simulink model "updated_target_driver_2026_withVariants_MPC_andwlqp2"  (R2024b)
settings: Solver=FixedStepDiscrete  StartTime=0.0  StopTime=running_time  FixedStep=dt_s  RelTol=1e-3
values from neighbouring files (symbols this model uses):
  A = gamma_2*gamma_3*Thrust_desired    [force2voltage.m]
  a2_lb = -0.25    [target_driver_setup_2022_Ctrl_V_2_4.m]    (also in target_driver_setup_2022_Ctrl_V_2_4_geometric.m; target_driver_setup_mpc_12msdelay.m; target_driver_setup_mpc_andWLQP.m)
  a2_openloop = -0    (= 0)    [target_driver_setup_2022_Ctrl_V_2_4.m]    (also in target_driver_setup_2022_Ctrl_V_2_4_geometric.m; target_driver_setup_mpc_12msdelay.m; target_driver_setup_mpc_andWLQP.m)
  a2_ub = 0.25    [target_driver_setup_2022_Ctrl_V_2_4.m]    (also in target_driver_setup_2022_Ctrl_V_2_4_geometric.m; target_driver_setup_mpc_12msdelay.m; target_driver_setup_mpc_andWLQP.m)
  att_s = 500    [target_driver_setup_2022_Ctrl_V_2_4.m]    (also in target_driver_setup_2022_Ctrl_V_2_4_geometric.m; target_driver_setup_mpc_12msdelay.m; target_driver_setup_mpc_andWLQP.m)
  c_vertical = 0.70e-3    (= 0.0007)    [target_driver_setup_mpc_andWLQP.m]
  closedloop_flag = 1    [target_driver_setup_2022_Ctrl_V_2_4.m]    (also in target_driver_setup_2022_Ctrl_V_2_4_geometric.m = 0; target_driver_setup_mpc_12msdelay.m = 0; target_driver_setup_mpc_andWLQP.m = 0)
  delay = delay-vicon_sample_cycle/2    [target_driver_setup_2022_Ctrl_V_2_4.m]    (also in target_driver_setup_2022_Ctrl_V_2_4_geometric.m; target_driver_setup_mpc_12msdelay.m; target_driver_setup_mpc_andWLQP.m)
  drv_amp = abs((vleft_p2p-vright_p2p))/2+min(vleft_p2p,vright_p2p)    [Wing_traj_to_Voltage.m]    (also in force2voltage.m; target_driver_setup_2022_Ctrl_V_2_4.m = 300; target_driver_setup_2022_Ctrl_V_2_4_geometric.m = 110; target_driver_setup_mpc_12msdelay.m = 150)
  drv_bias = max_drv_bias    (= 300)    [target_driver_setup_2022_Ctrl_V_2_4.m]    (also in target_driver_setup_2022_Ctrl_V_2_4_geometric.m = 200; target_driver_setup_mpc_12msdelay.m = 200; target_driver_setup_mpc_andWLQP.m = 200)
  drv_pitch_left = vleft_pitch    [Wing_traj_to_Voltage.m]    (also in force2voltage.m = 0; target_driver_setup_2022_Ctrl_V_2_4.m = 0; target_driver_setup_2022_Ctrl_V_2_4_geometric.m = 9.05; target_driver_setup_mpc_12msdelay.m = 9.05)
  drv_pitch_right = vright_pitch    [Wing_traj_to_Voltage.m]    (also in force2voltage.m = 0; target_driver_setup_2022_Ctrl_V_2_4.m = 0; target_driver_setup_2022_Ctrl_V_2_4_geometric.m = 9.05; target_driver_setup_mpc_12msdelay.m = 9.05)
  drv_roll = (vleft_p2p-vright_p2p)/4    [Wing_traj_to_Voltage.m]    (also in force2voltage.m; target_driver_setup_2022_Ctrl_V_2_4.m = 0; target_driver_setup_2022_Ctrl_V_2_4_geometric.m = -0.001; target_driver_setup_mpc_12msdelay.m = -0.001)
  dt_s = 1e-3    (= 0.001)    [target_driver_setup_2022_Ctrl_V_2_4.m]    (also in target_driver_setup_2022_Ctrl_V_2_4_geometric.m = 0.0002; target_driver_setup_mpc_12msdelay.m = 0.0002; target_driver_setup_mpc_andWLQP.m = 2.0e-4;1)
  f_fin = f    (= 180)    [target_driver_setup_2022_Ctrl_V_2_4.m]    (also in target_driver_setup_2022_Ctrl_V_2_4_geometric.m = 155; target_driver_setup_mpc_12msdelay.m = 155; target_driver_setup_mpc_andWLQP.m = 155)
  f_int = f    (= 180)    [target_driver_setup_2022_Ctrl_V_2_4.m]    (also in target_driver_setup_2022_Ctrl_V_2_4_geometric.m = 155; target_driver_setup_mpc_12msdelay.m = 155; target_driver_setup_mpc_andWLQP.m = 155)
  g = 9.8    [target_driver_setup_2022_Ctrl_V_2_4.m]    (also in target_driver_setup_2022_Ctrl_V_2_4_geometric.m; target_driver_setup_mpc_12msdelay.m; target_driver_setup_mpc_andWLQP.m = 9.81; test_full_attitude_mpc.m = 9.81)
  I_moment = eye(3)    [target_driver_exec_2022_Ctrl_V_2_4.m]    (also in target_driver_setup_2022_Ctrl_V_2_4.m; target_driver_setup_2022_Ctrl_V_2_4_geometric.m; target_driver_setup_mpc_12msdelay.m; target_driver_setup_mpc_andWLQP.m)
  k_tau_vec = [k_tau_roll;k_tau_pitch]    [target_driver_setup_2022_Ctrl_V_2_4_geometric.m]    (also in target_driver_setup_mpc_12msdelay.m; target_driver_setup_mpc_andWLQP.m)
  m = t <= t_zoom    [plot_roll_torque_cmd_vs_actual.m]    (also in plot_roll_torque_cmd_vs_actual_flightlog.m = t >= t0 & t <= t1; target_driver_setup_2022_Ctrl_V_2_4.m = 0.000124; target_driver_setup_2022_Ctrl_V_2_4_geometric.m = 8.5655e-05; target_driver_setup_mpc_12msdelay.m = 8.5655e-05)
  params_vec = [params_opt.delta_1, params_opt.delta_2, params_opt.delta_3,      params_opt.gamma_1, params_opt.gamma_2_1, params_opt.gamma_3,      params_opt.eta, params_opt.nu, params_opt.mu]'    [force2voltage_tuningSandbox.m]    (also in target_driver_setup_2022_Ctrl_V_2_4.m = [params_opt.delta_1, params_opt.delta_2, params_opt.delta_3,; target_driver_setup_2022_Ctrl_V_2_4_geometric.m = [params_opt.delta_1, params_opt.delta_2, params_opt.delta_3,; target_driver_setup_mpc_12msdelay.m = [params_opt.delta_1, params_opt.delta_2, params_opt.delta_3,; target_driver_setup_mpc_andWLQP.m = [params_opt.delta_1, params_opt.delta_2, params_opt.delta_3,)
  phase = 0    [target_driver_setup_2022_Ctrl_V_2_4.m]    (also in target_driver_setup_2022_Ctrl_V_2_4_geometric.m; target_driver_setup_mpc_12msdelay.m; target_driver_setup_mpc_andWLQP.m)
  popts_flattened = popts.popts    [target_driver_setup_mpc_andWLQP.m]
  roll_offset_angle = 0    [target_driver_setup_2022_Ctrl_V_2_4.m]    (also in target_driver_setup_2022_Ctrl_V_2_4_geometric.m; target_driver_setup_mpc_12msdelay.m; target_driver_setup_mpc_andWLQP.m)
  running_time = start_delay+total_T    (= 9)    [target_driver_setup_2022_Ctrl_V_2_4.m]    (also in target_driver_setup_2022_Ctrl_V_2_4_geometric.m = 10; target_driver_setup_mpc_12msdelay.m = 0.5; target_driver_setup_mpc_andWLQP.m = 10)
  running_time_control = start_delay_control+total_T+0.0    (= 7.1)    [target_driver_setup_2022_Ctrl_V_2_4.m]    (also in target_driver_setup_2022_Ctrl_V_2_4_geometric.m = 10; target_driver_setup_mpc_12msdelay.m = 0.5; target_driver_setup_mpc_andWLQP.m = 10)
  sampling_f = 10000    [target_driver_setup_2022_Ctrl_V_2_4.m]    (also in target_driver_setup_2022_Ctrl_V_2_4_geometric.m = 5000; target_driver_setup_mpc_12msdelay.m = 5000; target_driver_setup_mpc_andWLQP.m = 1/dt_s)
  start_delay = 2.0    (= 2)    [target_driver_setup_2022_Ctrl_V_2_4.m]    (also in target_driver_setup_2022_Ctrl_V_2_4_geometric.m = 0; target_driver_setup_mpc_12msdelay.m = 0; target_driver_setup_mpc_andWLQP.m = 0)
  start_delay_control = start_delay + ramp_delay    (= 0.1)    [target_driver_setup_2022_Ctrl_V_2_4.m]    (also in target_driver_setup_2022_Ctrl_V_2_4_geometric.m = 0; target_driver_setup_mpc_12msdelay.m = 0; target_driver_setup_mpc_andWLQP.m = 0)
  T = 1    [target_driver_setup_2022_Ctrl_V_2_4.m]    (also in target_driver_setup_2022_Ctrl_V_2_4_geometric.m = 10; target_driver_setup_mpc_12msdelay.m = 0.5; target_driver_setup_mpc_andWLQP.m = 10; test_full_attitude_mpc.m = T0 + nu(1))
  weights_vec = [ws; wds; wpr_xy;wpr_z; wpf; wvr_xy; wvr_z ... (first row only)    [target_driver_setup_2022_Ctrl_V_2_4_geometric.m]    (also in target_driver_setup_mpc_12msdelay.m; target_driver_setup_mpc_andWLQP.m)
undefined symbols (not defined in the file or in its folder): Com1, ctrl_Ts, DiscIntNeverNeededParam, dspblkCoreblockFVToolHelper, gcbh, left_mapping, left_mapping_F_to_Phi, lp_den, lp_num, none, right_mapping, right_mapping_F_to_Phi
libraries: simulink x17, xpcseriallib x2, cstblocks x1, xpcnilib x1, xpcutilitieslib x1
(part 4 of 4)

== matlab function updated_target_driver_2026_withVariants_MPC_andwlqp2/Observer for averaged system1/Attitude Observer/Geometric derivative in SO(3)/First order geometric derivative in SO(3)  ==
  data: R_prev input; omega output size=[3 1]; R_cur input; omega_prev input; update input; count input; sampling_f input
function omega  = fcn(R_prev, R_cur, omega_prev, update, count,sampling_f)

Rot_cur = [R_cur(1), R_cur(2), R_cur(3); R_cur(4), R_cur(5), R_cur(6); R_cur(7), R_cur(8), R_cur(9)];
Rot_prev = [R_prev(1), R_prev(2), R_prev(3); R_prev(4), R_prev(5), R_prev(6); R_prev(7), R_prev(8), R_prev(9)];

R_diff = Rot_prev'*Rot_cur;

tr_R_diff = trace(R_diff);
omega = zeros(3,1);
if update>0
   omega=omega_prev; 
else
    
% isreal(tr_R_diff)
if abs((tr_R_diff-1)/2)<=1
    theta = acos((tr_R_diff-1)/2);
else
    theta=acos((tr_R_diff-1)/2/abs((tr_R_diff-1)/2));
end

% To avoid NaN for omega
if theta<1e-10
	omega = omega_prev;
else
	w = 1/(2*sin(theta))*[R_diff(3,2)-R_diff(2,3); R_diff(1,3) - R_diff(3,1); R_diff(2,1)-R_diff(1,2)];

	omega = w*theta*sampling_f/(count+1);
end   

end
% 
% if theta==0 %update~=0 
%     y = y_prev;
% else
%      w = 1/(2*sin(theta))*[R_diff(3,2)-R_diff(2,3); R_diff(1,3) - R_diff(3,1); R_diff(2,1)-R_diff(1,2)];
%      y = w*theta*10000/20;
% end

== matlab function updated_target_driver_2026_withVariants_MPC_andwlqp2/Observer for averaged system1/Euler derivative & filtered angular velocity /Angular velocity ==
  data: R input; Rdot input; w output; Frob_error output
function [w,Frob_error] = fcn(R,Rdot)
%#codegen
Rot = [R(1), R(2), R(3); R(4), R(5), R(6); R(7), R(8), R(9); ];
dRot = [Rdot(1), Rdot(2), Rdot(3); Rdot(4), Rdot(5), Rdot(6); Rdot(7), Rdot(8), Rdot(9); ];

A = Rot'*dRot;
w_hat = 1/2*(A-A');
w=zeros(3,1);
w(1) = w_hat(3,2);
w(2) = w_hat(1,3);
w(3) = w_hat(2,1);
% wz = w(3);
Frob_error=trace((A+A')*(A+A'));

== matlab function updated_target_driver_2026_withVariants_MPC_andwlqp2/Observer for averaged system1/Position Observer/Averaging position & velocity  ==
  data: r_prev input; r_prev2 input; r_prev3 input; r_cur input; update input; count input; rout_prev input; rout output; vout_prev input; vout output; sampling_f input
function [rout, vout] = fcn(r_prev,r_prev2,r_prev3,r_cur,update, count,rout_prev,vout_prev,sampling_f)
%#codegen

rout = zeros(3,1);
vout = zeros(3,1);
if update>0
   rout=rout_prev; 
   vout=vout_prev;
else

    % 1 cycle average
    n= 4;
    
    rout = (r_prev+r_prev2+r_prev3+r_cur)/n;
    vout = (rout-rout_prev)*sampling_f/(count+1);
    
  
end

end

== matlab function updated_target_driver_2026_withVariants_MPC_andwlqp2/Vicon Post Processing1/Vicon Validity check/MATLAB Function3 ==
  data: R_prev input; y output; R_cur input
function y = fcn(R_prev,R_cur)
Rot_cur = [R_cur(1), R_cur(2), R_cur(3); R_cur(4), R_cur(5), R_cur(6); R_cur(7), R_cur(8), R_cur(9)];
Rot_prev = [R_prev(1), R_prev(2), R_prev(3); R_prev(4), R_prev(5), R_prev(6); R_prev(7), R_prev(8), R_prev(9)];

A=Rot_cur'*Rot_prev;
epsilonn = 1e-18;

if trace((A-eye(3))'*(A-eye(3)))<epsilonn
   y=0; 
else
    y=1;
end

== matlab function updated_target_driver_2026_withVariants_MPC_andwlqp2/Vicon Post Processing1/Vicon correction ==
  data: R_cur input; Rot_corrected_vec output; roll_offset_angle input
function Rot_corrected_vec = fcn(R_cur,roll_offset_angle)

Rot_cur = [R_cur(1), R_cur(2), R_cur(3); R_cur(4), R_cur(5), R_cur(6); R_cur(7), R_cur(8), R_cur(9)];
Rot_correction = [1, 0, 0; ...
									0, cos(roll_offset_angle), -sin(roll_offset_angle);...
									0, sin(roll_offset_angle), cos(roll_offset_angle)];
Rot_corrected = Rot_correction*Rot_cur;

Rot_corrected_vec = [Rot_corrected(1,1); Rot_corrected(1,2); Rot_corrected(1,3); Rot_corrected(2,1); Rot_corrected(2,2); Rot_corrected(2,3); Rot_corrected(3,1); Rot_corrected(3,2); Rot_corrected(3,3)];

end

== matlab function updated_target_driver_2026_withVariants_MPC_andwlqp2/Vicon correction1 ==
  data: x_cur input; x_corrected_vec output; roll_offset_angle input
function x_corrected_vec = fcn(x_cur,roll_offset_angle)

x_cur_vec = [x_cur(1); x_cur(2); x_cur(3)];
Rot_correction = [1, 0, 0; ...
									0, cos(roll_offset_angle), -sin(roll_offset_angle);...
									0, sin(roll_offset_angle), cos(roll_offset_angle)];
x_corrected_vec = Rot_correction*x_cur_vec;

end

== matlab function updated_target_driver_2026_withVariants_MPC_andwlqp2/Open_Closed_loop_selection/MATLAB Function ==
  data: time input; freq output; f_int parameter; f_fin parameter; T parameter
function freq = fcn(time, f_int, f_fin, T)
%#codegen

freq = f_int;
buffer_t = 0.0; %3.0
rel_time = time-buffer_t;
if rel_time > 0
    freq = f_int + (f_fin-f_int) * (rel_time/T);
end

if freq > f_fin
    freq = f_fin;
end

== matlab function updated_target_driver_2026_withVariants_MPC_andwlqp2/Force to voltage/Control Mode/Desired_Force_to_Voltage ==
  data: Thrust_desired input; drv_amp output; Roll_torque_desired input; Pitch_torque_desired input; Yaw_torque_desired input; drv_roll output; drv_pitch_left output; drv_pitch_right output; a2_coeff output; params_vec input
function [drv_amp, drv_roll, drv_pitch_left, drv_pitch_right, a2_coeff] =    fcn(Thrust_desired, Roll_torque_desired, Pitch_torque_desired, Yaw_torque_desired, params_vec)

% 
% Thrust_desired = 0.7e-3;% N
% Roll_torque_desired = 20e-6; %mN mm 
% Pitch_torque_desired = 0;% N  
% Yaw_torque_desired = 0;  
[drv_amp, drv_roll, drv_pitch_left, drv_pitch_right, a2_coeff] = force2voltage( ...
    Thrust_desired, Roll_torque_desired, Pitch_torque_desired, ...
    Yaw_torque_desired, params_vec);
% % global params_opt
% 
% delta_1 = params_vec(1);
% delta_2 = params_vec(2);
% delta_3 = params_vec(3);
% gamma_1 = params_vec(4);
% gamma_2 = params_vec(5);
% gamma_3 = params_vec(6);
% eta = params_vec(7);
% nu = params_vec(8);
% mu = params_vec(9);
% 
% 
% % Initializing for averaging filter at the end to prevent InF
% if Thrust_desired==0    
%     u4 = 0;
% else
%     u4 = Pitch_torque_desired/(Thrust_desired*delta_3*gamma_2)-nu;
% end
% 
% 
% % u3 calculation when tau approaches to zero
% if abs(Yaw_torque_desired)<1e-12
% 
%    u3 = -mu;
% else
%     % Bounds for the mapping to produce real solution
%     lb =(Thrust_desired/2)*(gamma_2*gamma_3*delta_2*mu/delta_1-sqrt((gamma_2*gamma_3*delta_2*Thrust_desired*mu/delta_1)^2+gamma_2*gamma_3));
%     ub =(Thrust_desired/2)*(gamma_2*gamma_3*delta_2*mu/delta_1+sqrt((gamma_2*gamma_3*delta_2*Thrust_desired*mu/delta_1)^2+gamma_2*gamma_3));
% 
%     if Yaw_torque_desired>=ub
%        Yaw_torque_desired = ub;
%     elseif Yaw_torque_desired<=lb
%        Yaw_torque_desired = lb; 
%     end
% 
%     % u3 calculation when tau approaches zero
%     if abs(Yaw_torque_desired) < 1e-12
%         u3 = -mu;
%     else
%         A = gamma_2*gamma_3*Thrust_desired;
%         B = gamma_2*gamma_3*delta_2*Thrust_desired*mu/delta_1;
% 
%         disc = A^2 - 4*Yaw_torque_desired*(Yaw_torque_desired - B);
% 
%     % Numerical / feasibility guard
%     if disc < 0
%         disc = 0;
%     end
% 
%     u3 = delta_1*(A - sqrt(disc))/(2*delta_2*Yaw_torque_desired);
%     end
% end
% 
% D = delta_1^2+delta_2^2*u3^2;
% % gamma_2*Thrust_desired+Roll_torque_desired 
% u1 = (gamma_2*Thrust_desired+Roll_torque_desired)/(2*gamma_1*gamma_2*D*eta);
% u2 = (gamma_2*Thrust_desired-Roll_torque_desired)/(2*gamma_1*gamma_2*D);
% 
% u1 = max(u1, 0); 
% u2 = max(u2, 0); % Guard against negative voltage
% vleft_p2p = sqrt(u1)*2; 
% vright_p2p = sqrt(u2)*2;
% vleft_pitch = u4;
% vright_pitch = u4;
% 
% 
% drv_amp = abs((vleft_p2p-vright_p2p))/2+min(vleft_p2p,vright_p2p); % p2p
% drv_roll = (vleft_p2p-vright_p2p)/4; % Amplitude
% drv_pitch_left = vleft_pitch;
% drv_pitch_right = vright_pitch;
% a2_coeff = u3;
% 
end

== matlab function updated_target_driver_2026_withVariants_MPC_andwlqp2/WLQP ==
  data: u0 input size=4; pdotdes input size=6; u output size=4; h0 input size=6; popts input size=90; controlRate input size=1; umin input size=4; umax input size=4; dumax input size=4; Qdiag input size=6; w0 output size=6; wrenchBias input
function [u, w0] = fcn(u0, pdotdes, h0, popts, controlRate, umin, umax, dumax, Qdiag, wrenchBias)
%#codegen
    % wrenchBias = wrenchBias * 0; 
    % One-wingbeat moving average on the MPC request (32 samples = 6.4 ms at
    % 5 kHz / 155 Hz). Exact nulls at 155 Hz and its harmonics, which is where
    % 86% of the pitch-request power sits (ff27). Without it the WLQP rate
    % limits clip the chatter asymmetrically and over-deliver ~0.01 mN of lift.
    N_MA = 32;
    persistent buf idx
    if isempty(buf)
        buf = zeros(6, N_MA);
        idx = 1;
    end
    buf(:, idx) = pdotdes;
    idx = idx + 1;
    if idx > N_MA
        idx = 1;
    end
    pdotdes_f = sum(buf, 2) / N_MA;

    [u, w0] = wlqp(u0, pdotdes, h0, popts, controlRate, umin, umax, dumax, Qdiag, wrenchBias); 
end

== matlab function updated_target_driver_2026_withVariants_MPC_andwlqp2/Open_Closed_loop_selection/MATLAB Function4 ==
  data: openloop_control input; closedloop_control input; drv_amp_final output; closedloop_flag input; drv_pch_final_left output; drv_pch_final_right output; drv_roll_final output; a2_final output
function [drv_amp_final, drv_pch_final_left,drv_pch_final_right, drv_roll_final, a2_final] = fcn(openloop_control, closedloop_control, closedloop_flag)

if closedloop_flag==1
    drv_amp_final =closedloop_control(1);
    drv_pch_final_left =closedloop_control(2);
		drv_pch_final_right =closedloop_control(3);
    drv_roll_final=closedloop_control(4);
		a2_final=closedloop_control(5);
else
    drv_amp_final =openloop_control(1);
    drv_pch_final_left =openloop_control(2);
		drv_pch_final_right =openloop_control(3);
    drv_roll_final=openloop_control(4);
		a2_final=openloop_control(5);
		
end

== matlab function updated_target_driver_2026_withVariants_MPC_andwlqp2/Variant Subsystem/Simulation/MATLAB Function ==
  data: time output; dt_s input; left_voltage_v input; right_voltage_v input; bias_voltage_v input; x output; y output; z output; alpha_rad output; beta_rad output; gamma_rad output
function [time,x,y,z,alpha_rad,beta_rad,gamma_rad] = fcn(dt_s, left_voltage_v, right_voltage_v, bias_voltage_v)
%#codegen

pose = robobee_tcp_step_codegen(dt_s, left_voltage_v, right_voltage_v, bias_voltage_v);

time      = pose(1);
x         = pose(2);
y         = pose(3);
z         = pose(4);
alpha_rad = pose(5);
beta_rad  = pose(6);
gamma_rad = pose(7);

end

== matlab function updated_target_driver_2026_withVariants_MPC_andwlqp2/MATLAB Function ==
  data: t input; pdes output; pos0 input; trajFreq input; trajAmp input; dpdes output; sdes output; pdes_log output; aref output; yaw_ref output
function [pdes, dpdes, sdes, pdes_log, aref, yaw_ref] = desTraj(t, pos0, trajFreq, trajAmp)
%#codegen
% Trajectory reference generator. MODE selects:
%   0  hover-hold at pos0
%   1  helix: circle (trajAmp radius, trajFreq Hz) about pos0 + climb,
%      spiral-out ramp, exact dpdes and aref (see helix comments below)
%   2  flip: hold position, schedule sdes through FLIP_FRACTION of a full
%      rotation about the roll axis (flight_tasks.py flip(), made C^2)
%   3  transit: straight line from pos0 to GOTO_TARGET, trapezoidal
%      (auto-triangular) velocity profile. sdes is NOT upright: it points
%      along the required specific force aref + g*e3 + K_DRAG*dpdes, so
%      the ws cost pulls the vehicle INTO the tilt forward flight needs
%      (flapping counter-force makes cruise at v require sustained tilt;
%      upright sdes fights it and caps speed -- see pitch-trim ceiling).
%   4  yaw spin: hold position at pos0, upright, and rotate the heading
%      reference about world z at SPIN_RATE (smootherstep ramp in/out).
%      Isolates the yaw loop: no translation, so nothing else changes.
%   5  centre-facing orbit, in phases: (a) take off and hover at pos0 for
%      T_ORBIT_START; (b) smootherstep transit over T_ORBIT_TRANSIT to the
%      orbit start point CENTER + R*[cos(THETA0); sin(THETA0); 0]; (c) pause
%      there T_ORBIT_PAUSE; (d) orbit ORBIT_CENTER at radius ORBIT_RADIUS,
%      period ORBIT_PERIOD, rate ramped in over T_ORBIT_RAMP (smootherstep,
%      exact integral as in mode 4). Body-x points at the centre THROUGHOUT
%      (psi = orbit angle + pi, dpsi = orbit rate). The centre sits AHEAD
%      of the start point (THETA0 = pi), so facing it is heading 0: the
%      hover and the +x transit are flown nose-first with NO yaw, and the
%      orbit begins from the heading the model starts with. On the orbit
%      the vehicle flies SIDEWAYS through body-y at 2*pi*R/T (0.063 m/s
%      for R 0.05, T 5): roll trim. sdes follows the specific force as in
%      mode 3.
%
% yaw_ref = [psi_des; dpsi_des; valid]  heading reference consumed by the
%   MPC yaw PID (upright_template_mpc_wl, HEADING_FOLLOW). psi_des is the
%   world heading of body-x [rad, wrapped], dpsi_des its rate [rad/s]
%   (feed-forward for the D term). valid = 0 tells the MPC to HOLD the
%   heading latched at engagement (old behaviour); valid = 1 to slew toward
%   psi_des. Modes 1 and 3 point body-x along the horizontal velocity
%   reference so the vehicle always flies FORWARD through the body frame:
%   with a fixed heading an orbit or lateral transit runs backward through
%   body-x, and the nose-up pitch trim that needs exceeds the +0.18 uoffs
%   box at ~0.27 m/s (failed_ellipse1: tumble at 3.64 s).
%
% FLIP PREREQUISITES -- read before setting MODE = 2:
%   * The current MPC has no ds_des (attitude-rate) reference: a rotating
%     sdes makes the wds cost fight the commanded rotation (this is what
%     destabilized the banked helix). A full flip needs the stage-varying
%     reference / LTV upgrade in upright_template_mpc_wl first.
%     Use FLIP_FRACTION <= 0.25 (90 deg excursion) to test incrementally.
%   * Altitude: during the rotation thrust cannot support weight; the bee
%     falls ~0.5*g*T_FLIP_DUR^2 plus recovery overshoot. Command pos0 z
%     >= 0.5 m before attempting large fractions.
%   * ds_des (for the future controller hookup) is analytically
%     ds_des = (2*pi*FLIP_FRACTION*phd) * [0; cos(ang); -sin(ang)].

MODE = 4;            % 0 hover | 1 helix | 2 flip | 3 transit | 4 yaw spin
                     % 5 centre-facing orbit

% ---- heading reference (modes 1, 3) ----
V_HEAD_MIN = 0.05;   % [m/s] horizontal |dpdes| below which heading holds

% ---- helix parameters ----
CLIMB_RATE = 0.0;   % [m/s] vertical rate of the helix
T_START    = 0.5;    % [s] hold at pos0 before the helix begins
T_RAMP     = 2.0;    % [s] radius/climb ramp-in duration

% ---- flip parameters ----
T_FLIP_START  = 1.0;   % [s] settle/hover time before the maneuver
T_FLIP_DUR    = 1.0;   % [s] duration of the scheduled rotation
FLIP_FRACTION = 1.0;  % fraction of a full turn: 0.25 = 90 deg out-and-
                       % back tilt test, 1.0 = full flip (needs LTV MPC)

% ---- transit parameters ----
GOTO_TARGET = [2.0; 0.0; 0.05]; % [m] target position
T_GOTO      = 0.75;              % [s] hover at pos0 before departure
V_CRUISE    = 0.9;              % [m/s] cruise speed (roll loop degrades
                                %       and pitch trim runs out ~0.5)
A_MAX       = 1.0;              % [m/s^2] accel/decel magnitude
c_x         = 7.14e-4;
K_DRAG      = 0.70e-3/(84.2e-6);   % [1/s] flapping counter-force c/m from
                                %       step ID; sets the cruise tilt
G_REF       = 9.81;             % [m/s^2]

% ---- yaw spin parameters ----
T_SPIN_START  = 0.5;      % [s] hover before the spin starts
T_SPIN_RAMP   = 0.1;      % [s] smootherstep ramp of the rate, in and out
SPIN_RATE     = 2*pi/5;       % [rad/s] plateau heading rate (+ = CCW seen from
                          %         above, i.e. +z). pi = one turn per 2 s.
                          %         Keep below the MPC's PSI_SLEW_MAX (6).
SPIN_DURATION = 4.0;      % [s] plateau duration before ramping back down
PSI_SPIN0     = 0.0;      % [rad] heading at spin start (model starts at 0;
                          %       the MPC slews from its latched heading to
                          %       this, so small mismatches are absorbed)

% ---- centre-facing orbit parameters (mode 5) ----
ORBIT_CENTER  = [0.10; 0.0; 0.05]; % [m] circle centre (world). Placed
                                  %       AHEAD of the start point so
                                  %       that facing the centre there is
                                  %       heading 0: no yaw during hover,
                                  %       transit or pause.
ORBIT_RADIUS  = 0.05;             % [m]
ORBIT_PERIOD  = 5.0;              % [s] one revolution
ORBIT_THETA0  = pi;               % [rad] start angle on the circle: the
                                  %       start point is CENTER + R*[cos;
                                  %       sin; 0] = [0.05; 0; 0.05], and
                                  %       heading = THETA0 + pi = 0 there
ORBIT_DIR     = +1.0;             % +1 CCW seen from above (+z), -1 CW
T_ORBIT_START   = 0.5;            % [s] hover at pos0 (take-off) first
T_ORBIT_TRANSIT = 1.0;            % [s] smootherstep move pos0 -> start
                                  %     point (0.05 m: 0.094 m/s peak,
                                  %     0.29 m/s^2 peak)
T_ORBIT_PAUSE   = 0.5;            % [s] hold at the start point before
                                  %     the orbit begins
T_ORBIT_RAMP    = 1.0;            % [s] smootherstep ramp of the orbit
                                  %     rate 0 -> 2*pi/ORBIT_PERIOD.
                                  %     Heading rate at plateau is
                                  %     1.26 rad/s: check tau_yaw_max.

p0 = reshape(double(pos0), 3, 1);
pdes  = p0;
dpdes = zeros(3,1);
aref  = zeros(3,1);
sdes  = [0; 0; 1];
yaw_ref = [0.0; 0.0; 0.0];       % default: hold latched heading

if MODE == 1
    % Helix: spiral out from p0, orbit radius trajAmp about p0, climb.
    % trajAmp = 0 or trajFreq = 0 reduces to hover-hold.
    r  = trajAmp(1);
    wc = 2*pi*trajFreq(1);
    tt = t(1) - T_START;
    if tt < 0, tt = 0; end
    if tt >= T_RAMP
        s = 1.0; sd = 0.0; sdd = 0.0;

        q = T_RAMP/2 + (tt - T_RAMP);
    else
        x   = tt / T_RAMP;
        s   = x*x*x*(10.0 - 15.0*x + 6.0*x*x);
        sd  = (30.0*x*x - 60.0*x*x*x + 30.0*x*x*x*x) / T_RAMP;
        sdd = (60.0*x - 180.0*x*x + 120.0*x*x*x) / (T_RAMP*T_RAMP);
        q   = T_RAMP * (2.5*x^4 - 3.0*x^5 + x^6);
    end
    th = wc * tt;
    c = cos(th); sn = sin(th);
    pdes = [p0(1) + s*r*c; p0(2) + s*r*sn; p0(3) + CLIMB_RATE*q];
    dpdes = [sd*r*c - s*r*wc*sn; sd*r*sn + s*r*wc*c; CLIMB_RATE*s];
    aref = [sdd*r*c - 2.0*sd*r*wc*sn - s*r*wc*wc*c; ...
            sdd*r*sn + 2.0*sd*r*wc*c - s*r*wc*wc*sn; ...
            CLIMB_RATE*sd];
    % bank feed-forward disabled pending a proper ds_des reference:
    % a rotating sdes with the MPC's implicit ds_des = 0 makes the wds
    % cost fight the orbit's required attitude rotation.
    sdes = [0; 0; 1];
    yaw_ref = headingFromVelocity(dpdes, aref, V_HEAD_MIN);

elseif MODE == 2
    % Flip about the ROLL axis (3x pitch's torque authority on this
    % plant, and stable open-loop damping). Position reference holds at
    % p0 throughout: the QP knows thrust cannot fight gravity mid-flip
    % and plans the fall + recovery.
    phr = (t(1) - T_FLIP_START) / T_FLIP_DUR;
    if phr < 0, phr = 0; elseif phr > 1, phr = 1; end
    ph  = phr*phr*phr*(10.0 - 15.0*phr + 6.0*phr*phr);  % smootherstep
    ang = 2*pi * FLIP_FRACTION * ph;
    sdes = [0; sin(ang); cos(ang)];
    % FLIP_FRACTION < 1: sdes goes out and STAYS at the tilted attitude;
    % for an out-and-back excursion test, mirror the phase:
    if FLIP_FRACTION < 0.999
        ang = 2*pi * FLIP_FRACTION * (1.0 - abs(2.0*ph - 1.0));
        sdes = [0; sin(ang); cos(ang)];
    end

elseif MODE == 3
    % Straight-line transit pos0 -> GOTO_TARGET, trapezoidal velocity
    % profile (auto-triangular when the distance is too short to reach
    % V_CRUISE).
    dvec = GOTO_TARGET - p0;
    D = norm(dvec);
    if D > 1.0e-6
        u = dvec / D;

        ta = V_CRUISE / A_MAX;      % nominal accel duration
        da = 0.5*A_MAX*ta^2;        % distance covered accelerating
        if 2.0*da > D
            ta = sqrt(D/A_MAX);     % short trip: triangular profile
            vc = A_MAX*ta;
            tc = 0.0;
        else
            vc = V_CRUISE;
            tc = (D - 2.0*da)/vc;
        end

        tt = t(1) - T_GOTO;
        if tt <= 0.0                 % waiting to depart
            sp = 0.0; vp = 0.0; ap = 0.0;
        elseif tt < ta               % accelerating
            ap = A_MAX;
            vp = A_MAX*tt;
            sp = 0.5*A_MAX*tt^2;
        elseif tt < ta + tc          % cruising
            ap = 0.0;
            vp = vc;
            sp = 0.5*A_MAX*ta^2 + vc*(tt - ta);
        elseif tt < 2.0*ta + tc      % decelerating
            td = tt - ta - tc;
            ap = -A_MAX;
            vp = vc - A_MAX*td;
            sp = 0.5*A_MAX*ta^2 + vc*tc + vc*td - 0.5*A_MAX*td^2;
        else                         % arrived
            ap = 0.0; vp = 0.0; sp = D;
        end

        pdes  = p0 + u*sp;
        dpdes = u*vp;
        aref  = u*ap;

        % Heading: the transit direction is known before departure, so
        % point body-x along it from t = 0 (the yaw happens during the
        % T_GOTO hover instead of while already moving sideways), and keep
        % it after arrival. Horizontal component only; a purely vertical
        % transit holds the latched heading.
        if u(1)*u(1) + u(2)*u(2) > 1.0e-6
            yaw_ref = [atan2(u(2), u(1)); 0.0; 1.0];
        end
    end

    % Desired orientation: NOT upright. Thrust must point along the total
    % specific force, and the flapping counter-force adds K_DRAG*v on top
    % of aref + g*e3 (cruise at 0.5 m/s => ~21 deg forward tilt). An
    % upright sdes would make the ws cost fight exactly that tilt.
    f_orientation = aref + [0; 0; G_REF] + K_DRAG*dpdes;
    sdes = f_orientation / max(norm(f_orientation), 1.0e-9);

elseif MODE == 4
    % Yaw spin at hover. Rate profile: smootherstep up over T_SPIN_RAMP,
    % plateau SPIN_RATE for SPIN_DURATION, smootherstep down over
    % T_SPIN_RAMP, then hold. The angle is the exact integral of the rate
    % (integral of smootherstep s(x) is T*(2.5x^4 - 3x^5 + x^6)).
    tt = t(1) - T_SPIN_START;
    ang = 0.0; rate = 0.0;
    if tt > 0.0
        if tt < T_SPIN_RAMP                          % ramp up
            x = tt / T_SPIN_RAMP;
            rate = SPIN_RATE * x*x*x*(10.0 - 15.0*x + 6.0*x*x);
            ang  = SPIN_RATE * T_SPIN_RAMP * (2.5*x^4 - 3.0*x^5 + x^6);
        elseif tt < T_SPIN_RAMP + SPIN_DURATION      % plateau
            rate = SPIN_RATE;
            ang  = SPIN_RATE * (0.5*T_SPIN_RAMP + (tt - T_SPIN_RAMP));
        elseif tt < 2.0*T_SPIN_RAMP + SPIN_DURATION  % ramp down
            x = (tt - T_SPIN_RAMP - SPIN_DURATION) / T_SPIN_RAMP;
            rate = SPIN_RATE * (1.0 - x*x*x*(10.0 - 15.0*x + 6.0*x*x));
            ang  = SPIN_RATE * (0.5*T_SPIN_RAMP + SPIN_DURATION ...
                   + T_SPIN_RAMP * (x - (2.5*x^4 - 3.0*x^5 + x^6)));
        else                                         % done: hold
            rate = 0.0;
            ang  = SPIN_RATE * (T_SPIN_RAMP + SPIN_DURATION);
        end
    end
    psi = PSI_SPIN0 + ang;
    yaw_ref = [atan2(sin(psi), cos(psi)); rate; 1.0];

elseif MODE == 5
    % Centre-facing orbit in phases (see header). Orbit angle
    % th = THETA0 + DIR*ang(to), where ang is the exact integral of a
    % smootherstep-ramped rate (mode 4 algebra with SPIN_RATE -> wo and
    % no ramp-down) and to is the time since the orbit began.
    R  = ORBIT_RADIUS;
    wo = 2.0*pi / ORBIT_PERIOD;                   % [rad/s] orbit rate
    p_start = ORBIT_CENTER + R*[cos(ORBIT_THETA0); sin(ORBIT_THETA0); 0.0];
    tt = t(1) - T_ORBIT_START;                    % time since hover ended
    to = tt - T_ORBIT_TRANSIT - T_ORBIT_PAUSE;    % time since orbit began

    ang = 0.0; rate = 0.0; rated = 0.0;
    if tt <= 0.0
        % (a) hover at pos0 (take-off target)
        pdes  = p0;
    elseif tt < T_ORBIT_TRANSIT
        % (b) smootherstep transit pos0 -> p_start, exact derivatives
        x   = tt / T_ORBIT_TRANSIT;
        s   = x*x*x*(10.0 - 15.0*x + 6.0*x*x);
        sd  = (30.0*x*x - 60.0*x*x*x + 30.0*x*x*x*x) / T_ORBIT_TRANSIT;
        sdd = (60.0*x - 180.0*x*x + 120.0*x*x*x) / (T_ORBIT_TRANSIT*T_ORBIT_TRANSIT);
        dvec  = p_start - p0;
        pdes  = p0 + dvec*s;
        dpdes = dvec*sd;
        aref  = dvec*sdd;
    elseif to <= 0.0
        % (c) pause on the circle
        pdes  = p_start;
    else
        % (d) orbit, rate ramped in
        if to < T_ORBIT_RAMP
            x     = to / T_ORBIT_RAMP;
            rate  = wo * x*x*x*(10.0 - 15.0*x + 6.0*x*x);
            rated = wo * (30.0*x*x - 60.0*x*x*x + 30.0*x*x*x*x) / T_ORBIT_RAMP;
            ang   = wo * T_ORBIT_RAMP * (2.5*x^4 - 3.0*x^5 + x^6);
        else
            rate  = wo;
            rated = 0.0;
            ang   = wo * (0.5*T_ORBIT_RAMP + (to - T_ORBIT_RAMP));
        end
    end
    th   = ORBIT_THETA0 + ORBIT_DIR*ang;
    thd  = ORBIT_DIR*rate;
    thdd = ORBIT_DIR*rated;
    if to > 0.0
        c = cos(th); sn = sin(th);
        pdes  = ORBIT_CENTER + R*[c; sn; 0.0];
        dpdes = R*thd*[-sn; c; 0.0];
        aref  = R*thdd*[-sn; c; 0.0] - R*thd*thd*[c; sn; 0.0];
    end

    % Heading: body-x from the vehicle toward the centre = th + pi.
    psi = th + pi;
    yaw_ref = [atan2(sin(psi), cos(psi)); thd; 1.0];

    % Orientation along the required specific force (mode 3 reasoning);
    % at 0.063 m/s this is a ~3 deg lean toward the centre plus the drag
    % counter-tilt, small but consistent with the momentum model.
    f_orientation = aref + [0; 0; G_REF] + K_DRAG*dpdes;
    sdes = f_orientation / max(norm(f_orientation), 1.0e-9);
end

pdes_log = pdes;
end

function yaw_ref = headingFromVelocity(dpdes, aref, v_min)
% Body-x along the horizontal velocity reference; rate = d/dt atan2(vy,vx)
% = (vx*ay - vy*ax)/|v_xy|^2. Below v_min the heading is undefined: hold.
vh2 = dpdes(1)*dpdes(1) + dpdes(2)*dpdes(2);
if vh2 > v_min*v_min
    yaw_ref = [atan2(dpdes(2), dpdes(1)); ...
               (dpdes(1)*aref(2) - dpdes(2)*aref(1)) / vh2; ...
               1.0];
else
    yaw_ref = [0.0; 0.0; 0.0];
end
end
